simulink library "Battery_Unipi"  (R2015a)
settings: Solver=ode45  StartTime=0.0  StopTime=10.0  RelTol=1e-3
values from neighbouring files (symbols this model uses):
  Bp2 = [-1.5 1.5 7.5 15 30]    [cell_model_params.mat]
  Bp3 = [10 25 35]    [cell_model_params.mat]
  Cl = [29641.7999226 11503.9720666 12184.9115516 18949.1321111 29359.7546177 54435.9445363 17320.6503567 21800.5296599 11503.1153162 8402.73024324 12724.7029394 29641.7999226 ... (165 elements, 11x3x5)]    [cell_model_params.mat]
  Cs = [1794.38328245 1972.14957342 1304.6988008 2287.34411958 1394.94057765 2574.67200441 2711.54611884 2014.87350742 1837.29877376 1461.62116074 1549.27064076 1794.38328245 ... (165 elements, 11x3x5)]    [cell_model_params.mat]
  ENTROPY = [-0.0706337258527 -0.0545791979561 -0.0419765837168 -0.0287620517654 -0.0164740504248 -0.00302559167104 0.0100496853907 0.0236819820108 0.0382890628579 0.050946575251 0.063604087644 0.0768186195953 ... (50 elements, 50x1)]    [entropy.mat]
  N = 12    [cell_model_params.mat]
  ocv = [3.27067654763 3.32006132767 3.3625409396 3.37864461563 3.39474829166 3.41085196769 3.42695564372 3.44305931975 3.45916299578 3.4752666718 3.49137034783 3.50747402386 ... (101 elements, 1x101)]    [cell_model_params.mat]
  params_bp = [0 10 20 30 40 50 60 70 80 90 100]    [cell_model_params.mat]
  Rl = [0.00306579121698 0.00985095179058 0.015159872699 0.00697344374496 0.00685050473095 0.0168286148563 0.028842238204 0.00933556048236 0.00984564396619 0.0207825421227 0.0597713059702 0.00306579121698 ... (165 elements, 11x3x5)]    [cell_model_params.mat]
  Rs = [0.00681237649308 0.0137907776578 0.0142248736573 0.00670636858043 0.0102913336279 0.0171112771524 0.00861470287808 0.00777637938451 0.0115325080228 0.0160739212772 0.0270265485557 0.00681237649308 ... (165 elements, 11x3x5)]    [cell_model_params.mat]
  soc_bp = [0 1 2 3 4 5 6 7 8 9 10 11 ... (101 elements, 1x101)]    [cell_model_params.mat]
  SOC_EN = [0.199345854552 0.208169800236 0.215033250515 0.222873277857 0.22973569152 0.236601928766 0.244441497278 0.252282901109 0.26012751675 0.267965708772 0.275803900794 0.283643928136 ... (50 elements, 50x1)]    [entropy.mat]
undefined symbols (not defined in the file or in its folder): Cth, Ro, Rthca, Rthcc, SoC0, Ta
undefined symbols (not defined in the file): Qbattery, R0, SoCinitlut
libraries: simulink x18, Battery_Unipi x7, simulink_extras x2
settings Model: Creator=Rocco  LastModifiedBy=pc2

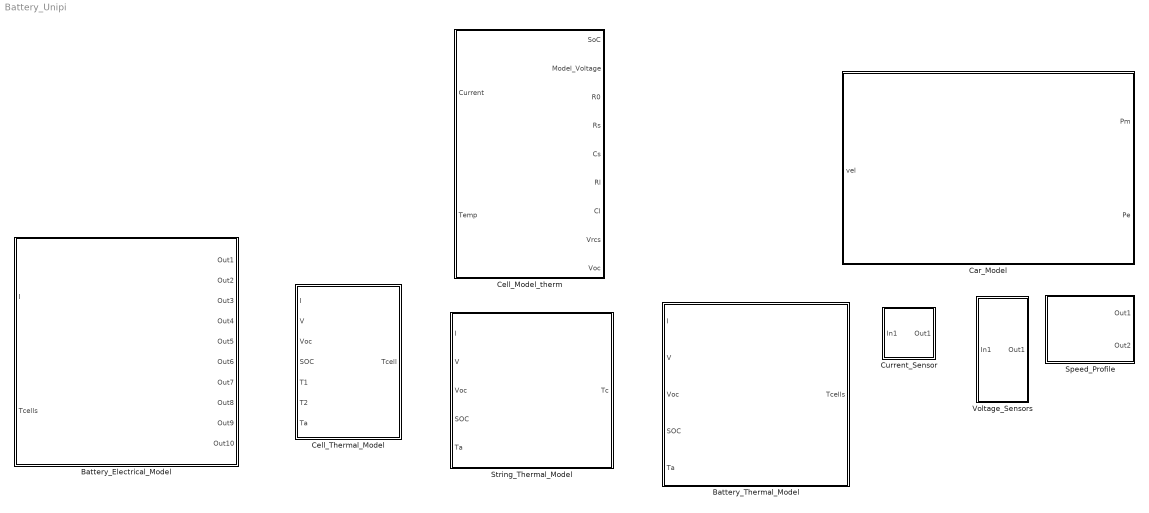
== system Battery_Unipi ==
  Battery_Electrical_Model : Subsystem  AncestorBlock=Battery_Unipi/Battery_Model_2  TreatAsAtomicUnit=on  mask{N=N, sampletime=sampletime, Qbattery=Qbattery, ocv=ocv, soc_bp=soc_bp, params_bp=params_bp, Ro=[repmat(R0,1,N)], Rs=[repmat(Rs,1,N)], Cs=[repmat(Cs,1,N)], Rl=[repmat(Rl,1,N)], Cl=[repmat(Cl,1,N)], SoC0=SoCinitlut, Bp2=Bp2, Bp3=Bp3}
      mask prompts: N "Number of cells"; sampletime "Sample time"; Qbattery "Battery Capacity (Coulomb)"; ocv "OCV-SOC LUT (101 points)"; soc_bp "OCV-SOC brakpoint (101points)"; params_bp "Parameter breackpoint (11 points)"; Ro "R0 (11 points)"; Rs "Rs (11 points)"; Cs "Cs (11 points)"; Rl "Rl (11 points)"; Cl "Cl (11 points)"; SoC0 "Initial SoC (%)"; Bp2 "Current breakpoint"; Bp3 "Temperature breakpoint"
      mask DialogControl DescTextVar Prompt: Battery composed of N series-connected cells. Each cell is modelled with an electric equivalent circuit with two RC groups. See Cell_Model block for more informations.
      mask DialogControl Control2 Prompt: Note: The OCV-SOC curve is the same for each cell.
      mask Display:
      | image('2013-9-3-5-7-21.jpg')
      | port_label('output', 1, 'SoCs')
      | port_label('output', 2, 'V_cells')
      | port_label('output', 3, 'R0')
      | port_label('output', 4, 'Rs')
      | port_label('output', 5, 'Cs')
      | port_label('output', 6, 'Rl')
      | port_label('output', 7, 'Cl')
      | port_label('output', 8, 'Vrcs')
      | port_label('output', 9, 'Voc')
      | port_label('output', 10, 'Vmcont')
      | port_label('input', 1, 'Current')
      | port_label('input', 2, 'Tcells')
  Battery_Thermal_Model : Subsystem  AncestorBlock=Battery_Unipi/Battery_Thermal_Model_obsolete  TreatAsAtomicUnit=on  mask{M=12, Rthca=Rthca, Rthcc=Rthcc, Cth=Cth, Ta=Ta, sampletime=sampletime}
      mask prompts: M "Number of cells into the string"; Rthca "Thermal resistance cell-to-ambient [K/W]"; Rthcc "Thermal resistance cell-to-cell [K/W]"; Cth "Thermal capacitance [J/W]"; Ta "Initial temperature [°C]"; sampletime "Sampletime [s]"
      mask DialogControl DescTextVar Prompt: Thermal model of a battery composed by a given number of series-connected cells, folded every M position
      mask Display:
      | image('therm.jpg')
      | port_label('output', 1, 'Tc')
      | port_label('input', 1, 'I')
      | port_label('input', 2, 'V')
      | port_label('input', 3, 'Voc')
      | port_label('input', 4, 'SOC')
      | port_label('input', 5, 'Ta')
  Car_Model : Subsystem  mask{M=1525, S=2.27, Cx=0.29, alphaR=0.01, roair=1.2, n_wheel=0.7, n_reg=0.5}
      mask prompts: M "Kerb weight (kg)"; S "Frontal area (m^2)"; Cx "Drag coefficient"; alphaR "Rolling resistance"; roair "Air density (kg m^-3)"; n_wheel "Efficiency battery->wheel"; n_reg "Efficiency wheel->battery"
      mask Display:
      | image('leaf.jpg')
      | port_label('output', 1, 'Pm')
      | port_label('output', 2, 'Pe')
      | port_label('input', 1, 'vel')
  Cell_Model_therm : Subsystem  AncestorBlock=Battery_Unipi/Cell_Model_therm  mask{Qn=Qbattery, ocv=ocv, soc_bp=soc_bp, params_bp=params_bp, R0=R0, Rs=Rs, Cs=Cs, Rl=Rl, Cl=Cl, Bp2=Bp2, Bp3=Bp3, SoC0=SoC0}
      mask prompts: Qn "Qn (Coulomb)"; ocv "OCV-SOC LUT (101 points)"; soc_bp "OCV-SOC breakpoint (101 points)"; params_bp "Parameter breakpoint (11 points)"; R0 "R0 (11 points)"; Rs "Rs (11 points)"; Cs "Cs (11 points)"; Rl "Rl (11 points)"; Cl "Cl (11 points)"; Bp2 "Current breakpoint"; Bp3 "Temperature breakpoint"; SoC0 "Initial SOC"
      mask DialogControl DescTextVar Prompt: Cell model with two RC groups
      mask Display:
      | image('unnamed.png')
      | port_label('output', 1, 'SoC')
      | port_label('output', 2, 'Vm')
      | port_label('output', 3, 'R0')
      | port_label('output', 4, 'Rs')
      | port_label('output', 5, 'Cs')
      | port_label('output', 6, 'Rl')
      | port_label('output', 7, 'Cl')
      | port_label('output', 8, 'Vrcs')
      | port_label('output', 9, 'Voc')
      | port_label('input', 1, 'Current')
      | port_label('input', 2, 'Temp')
  Cell_Thermal_Model : Subsystem  AncestorBlock=Battery_Unipi/cell_thermal_model  mask{Rthca=Rthca, Rthcc=Rthcc, Cth=Cth, Ta=24.833}
      mask prompts: Rthca "Thermal resistance cell-to-ambient [K/W]"; Rthcc "Thermal resistance cell-to-cell [K/W]"; Cth "Thermal capacitance [J/W]"; Ta "Initial temperature [°C]"
      mask Display:
      | image('big.png')
      | port_label('input', 1, 'I')
      | port_label('input', 2, 'V')
      | port_label('input', 3, 'Voc')
      | port_label('input', 4, 'SOC')
      | port_label('input', 5, 'T1')
      | port_label('input', 6, 'T2')
      | port_label('input', 7, 'Ta')
      | port_label('output', 1, 'Tc')
  Current_Sensor : Subsystem  mask{sampletime=sampletime, noisevariance=1, Offset=0, Nbits=16, FS=100}
      mask prompts: sampletime "Sample Time"; noisevariance "Variance"; Nbits "Number of bits"; FS "Full scale"
      mask DialogControl DescTextVar Prompt: This block is used to model the noise introduced by the current sensor and the ADC conversion
      mask Display: image('current_sensor.jpg')
  Speed_Profile : Subsystem  mask{selector=1}
      mask prompts: selector "Speed Profile"
      mask DialogControl DescTextVar Prompt: Select the speed test profile (1 for UDDS, 2 for HWFET, 3 for FTP, 4 for ECE_R15, 5 for EUDC, 6 for NEDC, 7 for WLTP_class_3, 8 for ArtUrban, 9 for ArtRoad, 10 for ArtMw130, 11 for ArtMw150, 12 for IM240, 13 for LA92, 14 for LA92short, 15 for NYCC, 16 for SFTP_SC03, 17 for SFTP_US06 and 18 for J1015).
      mask Display:
      | port_label('output', 1, 'Speed (km/h)')
      | port_label('output', 2, 'Speed (m/s)')
  String_Thermal_Model : Subsystem  AncestorBlock=Battery_Unipi/String_Thermal_Model_obsolete  mask{N=N, Rthca=Rthca, Rthcc=Rthcc, Cth=Cth, Ta=Ta, sampletime=sampletime}
      mask prompts: N "Number of cells"; Rthca "Thermal resistance cell-to-ambient [K/W]"; Rthcc "Thermal resistance cell-to-cell [K/W]"; Cth "Thermal capacitance [J/W]"; Ta "Initial temperature [°C]"; sampletime "Sampletime [s]"
      mask Display:
      | image('big_str.png')
      | port_label('output', 1, 'Tcell')
      | port_label('input', 1, 'I')
      | port_label('input', 2, 'V')
      | port_label('input', 3, 'Voc')
      | port_label('input', 4, 'SOC')
      | port_label('input', 5, 'Ta')
  Voltage_Sensors : Subsystem  mask{sampletime=0.1, noisevariance=1, Offset=0, Nbits=16, FS=5}
      mask prompts: sampletime "Sample Time"; noisevariance "Variance"; Nbits "Number of bits"; FS "Full scale"
      mask DialogControl DescTextVar Prompt: This block is used to model the noise introduced by the voltage sensor and the ADC conversion
      mask Display: image('ltc6804.jpg')

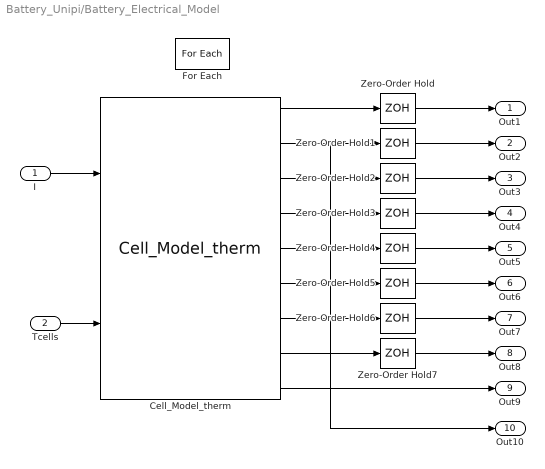
== system Battery_Unipi/Battery_Electrical_Model ==
  I : Inport  Partition=off
  Tcells : Inport  Port=2  Partition=on  PartitionDimension=1  PartitionWidth=1
  Cell_Model_therm : Battery_Unipi/Cell_Model_therm  Qn=Qbattery  ocv=ocv  soc_bp=soc_bp  params_bp=params_bp  R0=R0  Rs=Rs  Cs=Cs  Rl=Rl  Cl=Cl  Bp2=Bp2  Bp3=Bp3  SoC0=SoC0
  For Each : ForEach  DisableCoverage=on  IterateSubsysMaskParameter=off,off,on,off,off,off,on,on,on,on,on,on,off,off  SubsysMaskParameterIterationDimension=1,1,2,1,1,1,2,2,2,2,2,2,1,1  SubsysMaskParameterIterationStepSize=1,1,1,1,1,1,3,3,3,3,3,1,1,1  IndexMode=One-based
  Zero-Order Hold{,1..7} (8 alike) : ZeroOrderHold  SampleTime=sampletime
  Out1 : Outport  ConcatenationDimension=1
  Out2 : Outport  Port=2  ConcatenationDimension=1
  Out3 : Outport  Port=3  ConcatenationDimension=1
  Out4 : Outport  Port=4  ConcatenationDimension=1
  Out5 : Outport  Port=5  ConcatenationDimension=1
  Out6 : Outport  Port=6  ConcatenationDimension=1
  Out7 : Outport  Port=7  ConcatenationDimension=1
  Out8 : Outport  Port=8  ConcatenationDimension=1
  Out9 : Outport  Port=9  ConcatenationDimension=1
  Out10 : Outport  Port=10  ConcatenationDimension=1
  wires:
  Cell_Model_therm/9 -> Out9/1
  Tcells/1 -> Cell_Model_therm/2
  I/1 -> Cell_Model_therm/1
  Zero-Order Hold/1 -> Out1/1
  Cell_Model_therm/1 -> Zero-Order Hold/1
  Zero-Order Hold2/1 -> Out3/1
  Cell_Model_therm/3 -> Zero-Order Hold2/1
  Cell_Model_therm/2 -> Zero-Order Hold1/1, Out10/1
  Zero-Order Hold1/1 -> Out2/1
  Cell_Model_therm/7 -> Zero-Order Hold6/1
  Zero-Order Hold6/1 -> Out7/1
  Zero-Order Hold5/1 -> Out6/1
  Zero-Order Hold4/1 -> Out5/1
  Zero-Order Hold3/1 -> Out4/1
  Cell_Model_therm/4 -> Zero-Order Hold3/1
  Cell_Model_therm/5 -> Zero-Order Hold4/1
  Cell_Model_therm/6 -> Zero-Order Hold5/1
  Cell_Model_therm/8 -> Zero-Order Hold7/1
  Zero-Order Hold7/1 -> Out8/1

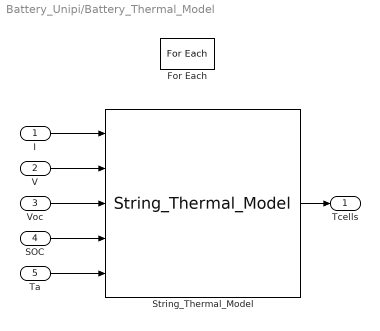
== system Battery_Unipi/Battery_Thermal_Model ==
  I : Inport  Partition=off
  V : Inport  Port=2  Partition=on  PartitionDimension=1  PartitionWidth=M
  Voc : Inport  Port=3  Partition=on  PartitionDimension=1  PartitionWidth=M
  SOC : Inport  Port=4  Partition=on  PartitionDimension=1  PartitionWidth=M
  Ta : Inport  Port=5  Partition=off
  For Each : ForEach  DisableCoverage=on  IndexMode=One-based
  String_Thermal_Model : Battery_Unipi/String_Thermal_Model  N=M  Rthca=Rthca  Rthcc=Rthcc  Cth=Cth  Ta=Ta  sampletime=sampletime
  Tcells : Outport  ConcatenationDimension=1
  wires:
  Ta/1 -> String_Thermal_Model/5
  V/1 -> String_Thermal_Model/2
  I/1 -> String_Thermal_Model/1
  String_Thermal_Model/1 -> Tcells/1
  Voc/1 -> String_Thermal_Model/3
  SOC/1 -> String_Thermal_Model/4

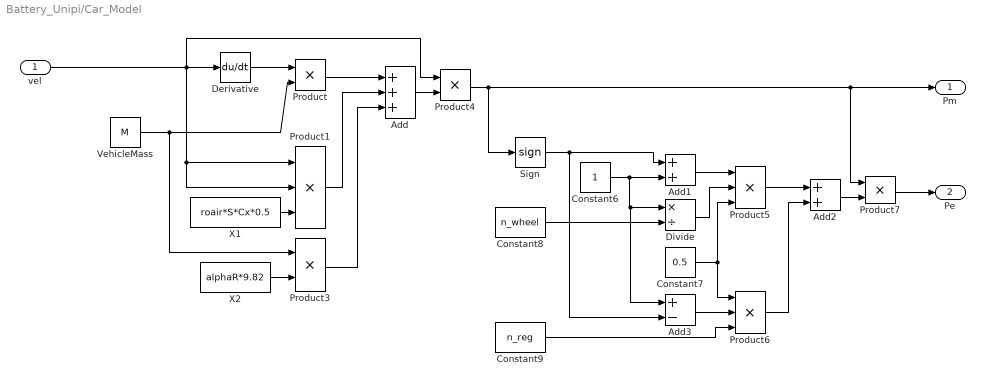
== system Battery_Unipi/Car_Model ==
  vel : Inport
  Add : Sum  Inputs=+++
  Add1 : Sum
  Add2 : Sum
  Add3 : Sum  Inputs=+-
  Constant6 : Constant
  Constant7 : Constant  Value=0.5
  Constant8 : Constant  Value=n_wheel
  Constant9 : Constant  Value=n_reg
  Derivative : Derivative
  Divide : Product  Inputs=*/
  Product{,3..4,7} (4 alike) : Product
  Product1 : Product  Inputs=3
  Product5 : Product  Inputs=3
  Product6 : Product  Inputs=3
  Sign : Signum  ZeroCross=off
  VehicleMass : Constant  Value=M
  X1 : Constant  Value=roair*S*Cx*0.5
  X2 : Constant  Value=alphaR*9.82
  Pm : Outport
  Pe : Outport  Port=2
  wires:
  Constant9/1 -> Product6/3
  Product/1 -> Add/1
  Add2/1 -> Product7/2
  Add3/1 -> Product6/2
  vel/1 -> Product4/1, Product1/2, Product1/1, Derivative/1
  VehicleMass/1 -> Product/2, Product3/1
  Product7/1 -> Pe/1
  Product3/1 -> Add/3
  Add/1 -> Product4/2
  Product5/1 -> Add2/1
  Constant7/1 -> Product6/1, Product5/3
  X2/1 -> Product3/2
  Add1/1 -> Product5/1
  Product4/1 -> Sign/1, Pm/1, Product7/1
  Sign/1 -> Add3/2, Add1/1
  Constant8/1 -> Divide/2
  Divide/1 -> Product5/2
  Product1/1 -> Add/2
  Constant6/1 -> Add3/1, Divide/1, Add1/2
  Derivative/1 -> Product/1
  Product6/1 -> Add2/2
  X1/1 -> Product1/3

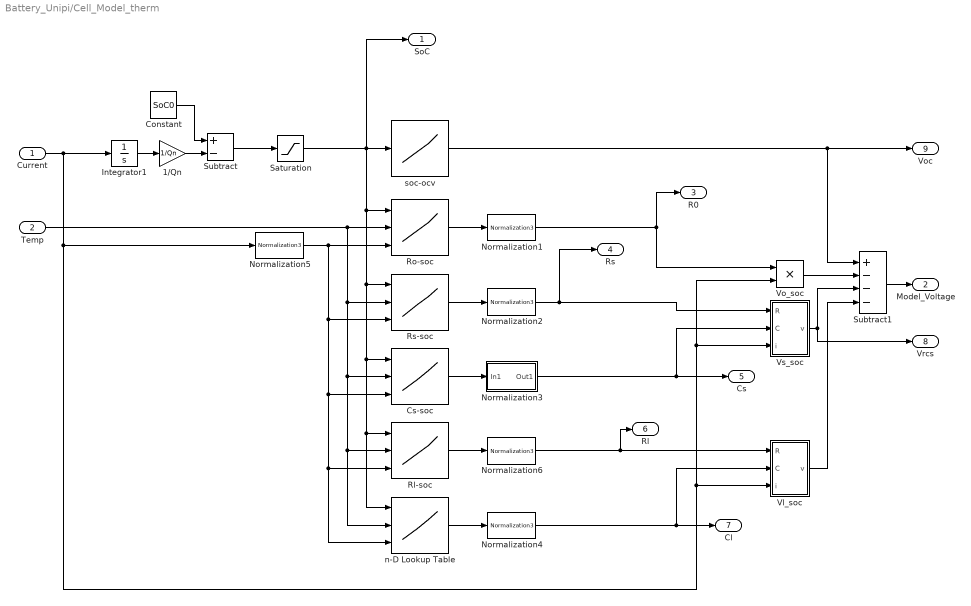
== system Battery_Unipi/Cell_Model_therm ==
  Current : Inport
  Temp : Inport  Port=2
  1/Qn : Gain  Gain=1/Qn
  Constant : Constant  Value=SoC0
  Cs-soc : Lookup_n-D  NumberOfTableDimensions=3  BreakpointsForDimension1=params_bp  BreakpointsForDimension2=Bp3  BreakpointsForDimension3=Bp2  Table=Cs  InterpMethod=Cubic spline  ExtrapMethod=Clip  UseLastTableValue=on  InternalRulePriority=Speed  RndMeth=Simplest  InputSameDT=on
  Integrator1 : Integrator
  Normalization1 : Battery_Unipi/Cell_Model_therm/Normalization3
      link override Constant3: Value=(1.5*3600)/Qn
  Normalization2 : Battery_Unipi/Cell_Model_therm/Normalization3
      link override Constant3: Value=(1.5*3600)/Qn
  Normalization3 : Subsystem  AncestorBlock=Battery_Unipi/Cell_Model/Normalization
  Normalization4 : Battery_Unipi/Cell_Model_therm/Normalization3
  Normalization5 : Battery_Unipi/Cell_Model_therm/Normalization3
      link override Constant3: Value=1.5/(Qn/3600)
  Normalization6 : Battery_Unipi/Cell_Model_therm/Normalization3
      link override Constant3: Value=(1.5*3600)/Qn
  Rl-soc : Lookup_n-D  NumberOfTableDimensions=3  BreakpointsForDimension1=params_bp  BreakpointsForDimension2=Bp3  BreakpointsForDimension3=Bp2  Table=Rl  InterpMethod=Cubic spline  ExtrapMethod=Clip  UseLastTableValue=on  InternalRulePriority=Speed  RndMeth=Simplest  InputSameDT=on
  Ro-soc : Lookup_n-D  NumberOfTableDimensions=3  BreakpointsForDimension1=params_bp  BreakpointsForDimension2=Bp3  BreakpointsForDimension3=Bp2  Table=Ro  InterpMethod=Cubic spline  ExtrapMethod=Clip  UseLastTableValue=on  InternalRulePriority=Speed  RndMeth=Simplest  InputSameDT=on
  Rs-soc : Lookup_n-D  NumberOfTableDimensions=3  BreakpointsForDimension1=params_bp  BreakpointsForDimension2=Bp3  BreakpointsForDimension3=Bp2  Table=Rs  InterpMethod=Cubic spline  ExtrapMethod=Clip  UseLastTableValue=on  InternalRulePriority=Speed  RndMeth=Simplest  InputSameDT=on
  Saturation : Saturate  UpperLimit=100  LowerLimit=0
  Subtract : Sum  Inputs=+-
  Subtract1 : Sum  Inputs=+---
  Vl_soc : Subsystem
  Vo_soc : Product
  Vs_soc : Subsystem
  n-D Lookup Table : Lookup_n-D  NumberOfTableDimensions=3  BreakpointsForDimension1=params_bp  BreakpointsForDimension2=Bp3  BreakpointsForDimension3=Bp2  Table=Cl  InterpMethod=Cubic spline  ExtrapMethod=Clip  UseLastTableValue=on  InternalRulePriority=Speed  RndMeth=Simplest  InputSameDT=on
  soc-ocv : Lookup_n-D  NumberOfTableDimensions=1  BreakpointsForDimension1=soc_bp  Table=ocv  InternalRulePriority=Speed  RndMeth=Simplest  InputSameDT=on
  SoC : Outport
  Model_Voltage : Outport  Port=2
  R0 : Outport  Port=3
  Rs : Outport  Port=4
  Cs : Outport  Port=5
  Rl : Outport  Port=6
  Cl : Outport  Port=7
  Vrcs : Outport  Port=8
  Voc : Outport  Port=9
  wires:
  Current/1 -> Integrator1/1, Normalization5/1, Vl_soc/3(i), Vs_soc/3(i), Vo_soc/2
  Normalization4/1 -> Vl_soc/2("C "), Cl/1
  Normalization3/1(Out1) -> Vs_soc/2("C "), Cs/1
  Normalization6/1 -> Vl_soc/1(R), Rl/1
  Normalization2/1 -> Vs_soc/1(R), Rs/1
  Normalization1/1 -> R0/1, Vo_soc/1
  Temp/1 -> Ro-soc/2, Rs-soc/2, n-D Lookup Table/2, Rl-soc/2, Cs-soc/2
  Subtract1/1 -> Model_Voltage/1
  Vo_soc/1 -> Subtract1/2
  Subtract/1 -> Saturation/1
  Constant/1 -> Subtract/1
  Vl_soc/1(v) -> Subtract1/4
  Vs_soc/1(v) -> Subtract1/3, Vrcs/1
  soc-ocv/1 -> Subtract1/1, Voc/1
  Rs-soc/1 -> Normalization2/1
  n-D Lookup Table/1 -> Normalization4/1
  Rl-soc/1 -> Normalization6/1
  Ro-soc/1 -> Normalization1/1
  Integrator1/1 -> 1/Qn/1
  Cs-soc/1 -> Normalization3/1(In1)
  1/Qn/1 -> Subtract/2
  Saturation/1 -> Ro-soc/1, Rs-soc/1, Cs-soc/1, Rl-soc/1, n-D Lookup Table/1, SoC/1, soc-ocv/1
  Normalization5/1 -> Ro-soc/3, n-D Lookup Table/3, Rl-soc/3, Cs-soc/3, Rs-soc/3

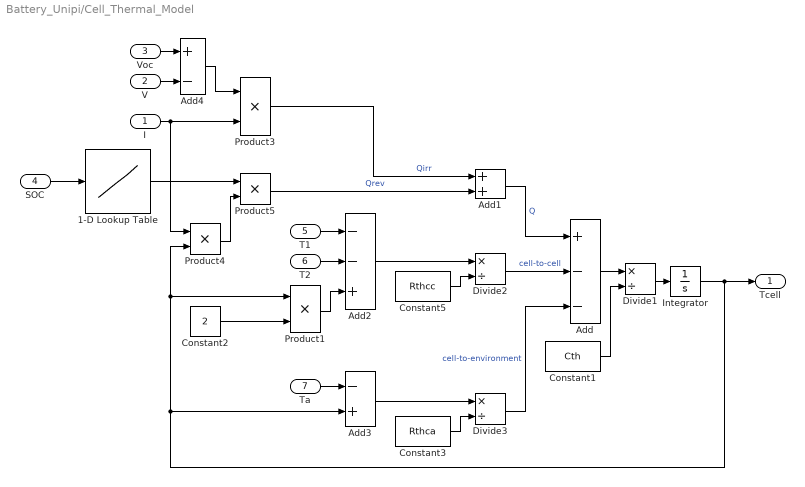
== system Battery_Unipi/Cell_Thermal_Model ==
  I : Inport
  V : Inport  Port=2
  Voc : Inport  Port=3
  SOC : Inport  Port=4
  T1 : Inport  Port=5
  T2 : Inport  Port=6
  Ta : Inport  Port=7
  1-D Lookup Table : Lookup_n-D  NumberOfTableDimensions=1  BreakpointsForDimension1=SOC_EN  BeginIndexSearchUsingPreviousIndexResult=on  Table=ENTROPY./1000  ExtrapMethod=Clip  UseLastTableValue=on  InternalRulePriority=Speed  RndMeth=Simplest  InputSameDT=on
  Add : Sum  Inputs=+--
  Add1 : Sum
  Add2 : Sum  Inputs=--+
  Add3 : Sum  Inputs=-+
  Add4 : Sum  Inputs=+-
  Constant1 : Constant  Value=Cth
  Constant2 : Constant  Value=2
  Constant3 : Constant  Value=Rthca
  Constant5 : Constant  Value=Rthcc
  Divide1 : Product  Inputs=*/
  Divide2 : Product  Inputs=*/
  Divide3 : Product  Inputs=*/
  Integrator : Integrator  InitialCondition=Ta
  Product{1,3..5} (4 alike) : Product
  Tcell : Outport
  wires:
  Integrator/1 -> Tcell/1, Product4/2, Product1/1, Add3/2
  I/1 -> Product3/2, Product4/1
  Add/1 -> Divide1/1
  Constant1/1 -> Divide1/2
  Divide1/1 -> Integrator/1
  Product4/1 -> Product5/2
  1-D Lookup Table/1 -> Product5/1
  SOC/1 -> 1-D Lookup Table/1
  Product3/1 -> Add1/1  "Qirr"
  Add1/1 -> Add/1  "Q"
  Constant2/1 -> Product1/2
  Product1/1 -> Add2/3
  T2/1 -> Add2/2
  T1/1 -> Add2/1
  Add2/1 -> Divide2/1
  Constant5/1 -> Divide2/2
  Divide2/1 -> Add/2  "cell-to-cell"
  Ta/1 -> Add3/1
  Constant3/1 -> Divide3/2
  Add3/1 -> Divide3/1
  Divide3/1 -> Add/3  "cell-to-environment"
  Product5/1 -> Add1/2  "Qrev"
  Add4/1 -> Product3/1
  Voc/1 -> Add4/1
  V/1 -> Add4/2

== system Battery_Unipi/Current_Sensor ==
  In1 : Inport
  Add : Sum
  Constant2 : Constant  Value=FS*2/(2^Nbits)
  Divide : Product  Inputs=**
  Idealized ADC quantizer : simulink_extras/Additional Discrete/Idealized ADC quantizer  NumberOfConverterBits=Nbits  Vmin=-FS  Vmax=FS  OutputDataType=single  OutputNegativeValues=on
  Noise : RandomNumber  Mean=Offset  Variance=noisevariance  SampleTime=sampletime
  Out1 : Outport
  wires:
  In1/1 -> Add/1
  Noise/1 -> Add/2
  Add/1 -> Idealized ADC quantizer/1
  Divide/1 -> Out1/1
  Idealized ADC quantizer/1 -> Divide/1
  Constant2/1 -> Divide/2

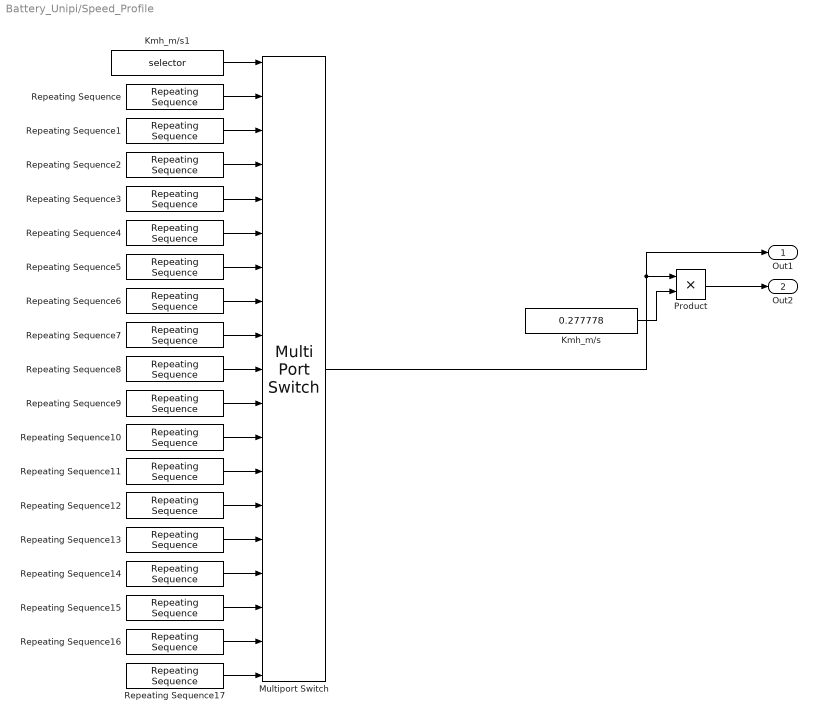
== system Battery_Unipi/Speed_Profile ==
  Kmh_m/s : Constant  Value=0.277778
  Kmh_m/s1 : Constant  Value=selector
  Multiport Switch : MultiPortSwitch  Inputs=18
  Product : Product
  Repeating Sequence : simulink/Sources/Repeating Sequence  rep_seq_t=UDDS.Time  rep_seq_y=UDDS.Data
  Repeating Sequence1 : simulink/Sources/Repeating Sequence  rep_seq_t=HWFET.Time  rep_seq_y=HWFET.Data
  Repeating Sequence10 : simulink/Sources/Repeating Sequence  rep_seq_t=ArtMw150.Time  rep_seq_y=ArtMw150.Data
  Repeating Sequence11 : simulink/Sources/Repeating Sequence  rep_seq_t=IM240.Time  rep_seq_y=IM240.Data
  Repeating Sequence12 : simulink/Sources/Repeating Sequence  rep_seq_t=LA92.Time  rep_seq_y=LA92.Data
  Repeating Sequence13 : simulink/Sources/Repeating Sequence  rep_seq_t=LA92short.Time  rep_seq_y=LA92short.Data
  Repeating Sequence14 : simulink/Sources/Repeating Sequence  rep_seq_t=NYCC.Time  rep_seq_y=NYCC.Data
  Repeating Sequence15 : simulink/Sources/Repeating Sequence  rep_seq_t=SFTP_SC03.Time  rep_seq_y=SFTP_SC03.Data
  Repeating Sequence16 : simulink/Sources/Repeating Sequence  rep_seq_t=SFTP_US06.Time  rep_seq_y=SFTP_US06.Data
  Repeating Sequence17 : simulink/Sources/Repeating Sequence  rep_seq_t=J1015.Time  rep_seq_y=J1015.Data
  Repeating Sequence2 : simulink/Sources/Repeating Sequence  rep_seq_t=FTP.Time  rep_seq_y=FTP.Data
  Repeating Sequence3 : simulink/Sources/Repeating Sequence  rep_seq_t=ECE_R15.Time  rep_seq_y=ECE_R15.Data
  Repeating Sequence4 : simulink/Sources/Repeating Sequence  rep_seq_t=EUDC.Time  rep_seq_y=EUDC.Data
  Repeating Sequence5 : simulink/Sources/Repeating Sequence  rep_seq_t=NEDC.Time  rep_seq_y=NEDC.Data
  Repeating Sequence6 : simulink/Sources/Repeating Sequence  rep_seq_t=WLTP_class_3.Time  rep_seq_y=WLTP_class_3.Data
  Repeating Sequence7 : simulink/Sources/Repeating Sequence  rep_seq_t=ArtUrban.Time  rep_seq_y=ArtUrban.Data
  Repeating Sequence8 : simulink/Sources/Repeating Sequence  rep_seq_t=ArtRoad.Time  rep_seq_y=ArtRoad.Data
  Repeating Sequence9 : simulink/Sources/Repeating Sequence  rep_seq_t=ArtMw130.Time  rep_seq_y=ArtMw130.Data
  Out1 : Outport
  Out2 : Outport  Port=2
  wires:
  Kmh_m/s1/1 -> Multiport Switch/1
  Repeating Sequence/1 -> Multiport Switch/2
  Repeating Sequence1/1 -> Multiport Switch/3
  Repeating Sequence2/1 -> Multiport Switch/4
  Repeating Sequence3/1 -> Multiport Switch/5
  Repeating Sequence4/1 -> Multiport Switch/6
  Repeating Sequence5/1 -> Multiport Switch/7
  Repeating Sequence6/1 -> Multiport Switch/8
  Repeating Sequence7/1 -> Multiport Switch/9
  Repeating Sequence8/1 -> Multiport Switch/10
  Repeating Sequence9/1 -> Multiport Switch/11
  Repeating Sequence10/1 -> Multiport Switch/12
  Kmh_m/s/1 -> Product/2
  Product/1 -> Out2/1
  Multiport Switch/1 -> Product/1, Out1/1
  Repeating Sequence11/1 -> Multiport Switch/13
  Repeating Sequence12/1 -> Multiport Switch/14
  Repeating Sequence13/1 -> Multiport Switch/15
  Repeating Sequence14/1 -> Multiport Switch/16
  Repeating Sequence15/1 -> Multiport Switch/17
  Repeating Sequence16/1 -> Multiport Switch/18
  Repeating Sequence17/1 -> Multiport Switch/19

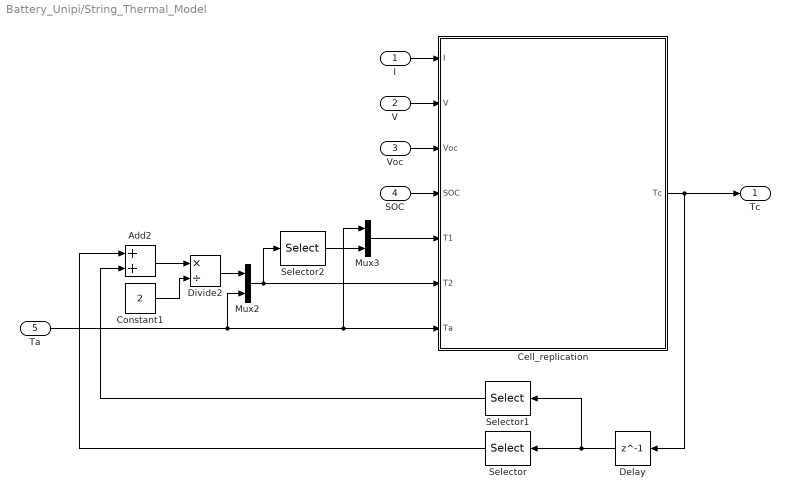
== system Battery_Unipi/String_Thermal_Model ==
  I : Inport
  V : Inport  Port=2
  Voc : Inport  Port=3
  SOC : Inport  Port=4
  Ta : Inport  Port=5
  Add2 : Sum
  Cell_replication : Subsystem  TreatAsAtomicUnit=on
  Constant1 : Constant  Value=2
  Delay : Delay  DelayLength=1  InitialCondition=0  SampleTime=sampletime
  Divide2 : Product  Inputs=*/
  Mux2 : Mux  Inputs=2
  Mux3 : Mux  Inputs=2
  Selector : Selector  NumberOfDimensions=2  InputPortWidth=N  IndexOptions=Index vector (dialog),Index vector (dialog)  Indices=[1:(N-1)],1  OutputSizes=1,1
  Selector1 : Selector  NumberOfDimensions=2  InputPortWidth=N  IndexOptions=Index vector (dialog),Index vector (dialog)  Indices=[2:N],1  OutputSizes=1,1
  Selector2 : Selector  NumberOfDimensions=2  InputPortWidth=N  IndexOptions=Index vector (dialog),Index vector (dialog)  Indices=[1:(N-1)],1  OutputSizes=1,1
  Tc : Outport
  wires:
  Delay/1 -> Selector1/1, Selector/1
  Cell_replication/1(Tc) -> Delay/1, Tc/1
  Selector/1 -> Add2/1
  V/1 -> Cell_replication/2(V)
  I/1 -> Cell_replication/1(I)
  Ta/1 -> Cell_replication/7(Ta), Mux3/1, Mux2/2
  Selector1/1 -> Add2/2
  Voc/1 -> Cell_replication/3(Voc)
  SOC/1 -> Cell_replication/4(SOC)
  Add2/1 -> Divide2/1
  Constant1/1 -> Divide2/2
  Divide2/1 -> Mux2/1
  Selector2/1 -> Mux3/2
  Mux2/1 -> Cell_replication/6(T2), Selector2/1
  Mux3/1 -> Cell_replication/5(T1)

== system Battery_Unipi/Voltage_Sensors ==
  In1 : Inport
  Add : Sum
  Constant : Constant  Value=FS/(2^Nbits)
  Divide : Product  Inputs=**
  Idealized ADC quantizer : simulink_extras/Additional Discrete/Idealized ADC quantizer  NumberOfConverterBits=Nbits  Vmin=0  Vmax=FS  OutputDataType=single  OutputNegativeValues=off
  Noise : RandomNumber  Mean=Offset  Variance=noisevariance  SampleTime=sampletime
  Out1 : Outport
  wires:
  In1/1 -> Add/1
  Noise/1 -> Add/2
  Idealized ADC quantizer/1 -> Divide/1
  Constant/1 -> Divide/2
  Add/1 -> Idealized ADC quantizer/1
  Divide/1 -> Out1/1

== system Battery_Unipi/Cell_Model_therm/Normalization3 ==
  In1 : Inport
  Constant3 : Constant  Value=(Qn/3600)/1.5
  Vo_soc1 : Product
  Out1 : Outport
  wires:
  Constant3/1 -> Vo_soc1/2
  Vo_soc1/1 -> Out1/1
  In1/1 -> Vo_soc1/1

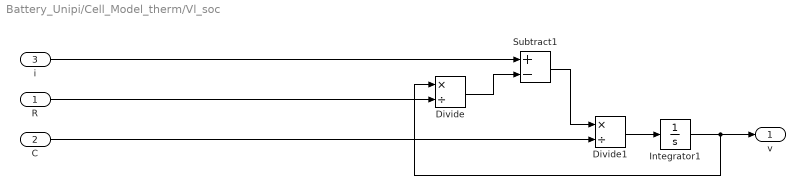
== system Battery_Unipi/Cell_Model_therm/Vl_soc ==
  R : Inport
  "C " : Inport  Port=2
  i : Inport  Port=3
  Divide : Product  Inputs=*/
  Divide1 : Product  Inputs=*/
  Integrator1 : Integrator  ContinuousStateAttributes='x1'
  Subtract1 : Sum  Inputs=+-
  v : Outport
  wires:
  "C "/1 -> Divide1/2
  R/1 -> Divide/2
  i/1 -> Subtract1/1
  Integrator1/1 -> v/1, Divide/1
  Divide1/1 -> Integrator1/1
  Subtract1/1 -> Divide1/1
  Divide/1 -> Subtract1/2

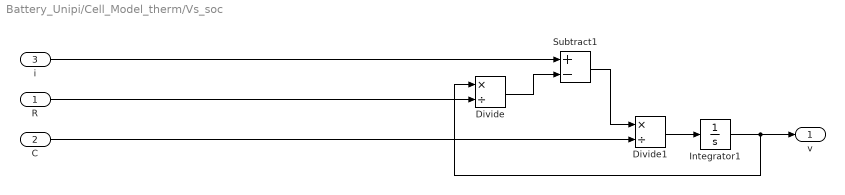
== system Battery_Unipi/Cell_Model_therm/Vs_soc ==
  R : Inport
  "C " : Inport  Port=2
  i : Inport  Port=3
  Divide : Product  Inputs=*/
  Divide1 : Product  Inputs=*/
  Integrator1 : Integrator
  Subtract1 : Sum  Inputs=+-
  v : Outport
  wires:
  R/1 -> Divide/2
  "C "/1 -> Divide1/2
  Integrator1/1 -> v/1, Divide/1
  Divide1/1 -> Integrator1/1
  Subtract1/1 -> Divide1/1
  i/1 -> Subtract1/1
  Divide/1 -> Subtract1/2

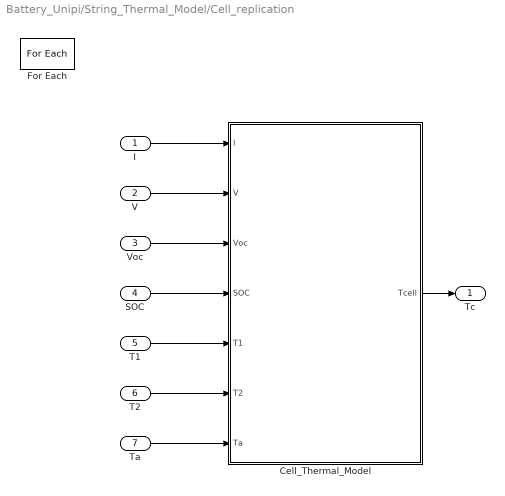
== system Battery_Unipi/String_Thermal_Model/Cell_replication ==
  I : Inport  Partition=off
  V : Inport  Port=2  Partition=on  PartitionDimension=1  PartitionWidth=1
  Voc : Inport  Port=3  Partition=on  PartitionDimension=1  PartitionWidth=1
  SOC : Inport  Port=4  Partition=on  PartitionDimension=1  PartitionWidth=1
  T1 : Inport  Port=5  Partition=on  PartitionDimension=1  PartitionWidth=1
  T2 : Inport  Port=6  Partition=on  PartitionDimension=1  PartitionWidth=1
  Ta : Inport  Port=7  Partition=off
  Cell_Thermal_Model : Subsystem  AncestorBlock=Battery_Unipi/cell_thermal_model  mask{Rthca=Rthca, Rthcc=Rthcc, Cth=Cth, Ta=Ta}
      mask prompts: Rthca "Thermal resistance cell-to-ambient [K/W]"; Rthcc "Thermal resistance cell-to-cell [K/W]"; Cth "Thermal capacitance [J/W]"; Ta "Initial temperature [°C]"
      mask Display:
      | image('big.png')
      | port_label('input', 1, 'I')
      | port_label('input', 2, 'V')
      | port_label('input', 3, 'Voc')
      | port_label('input', 4, 'SOC')
      | port_label('input', 5, 'T1')
      | port_label('input', 6, 'T2')
      | port_label('input', 7, 'Ta')
      | port_label('output', 1, 'Tc')
  For Each : ForEach  DisableCoverage=on  IndexMode=One-based
  Tc : Outport  ConcatenationDimension=1
  wires:
  T2/1 -> Cell_Thermal_Model/6(T2)
  T1/1 -> Cell_Thermal_Model/5(T1)
  Ta/1 -> Cell_Thermal_Model/7(Ta)
  V/1 -> Cell_Thermal_Model/2(V)
  I/1 -> Cell_Thermal_Model/1(I)
  Cell_Thermal_Model/1(Tcell) -> Tc/1
  Voc/1 -> Cell_Thermal_Model/3(Voc)
  SOC/1 -> Cell_Thermal_Model/4(SOC)

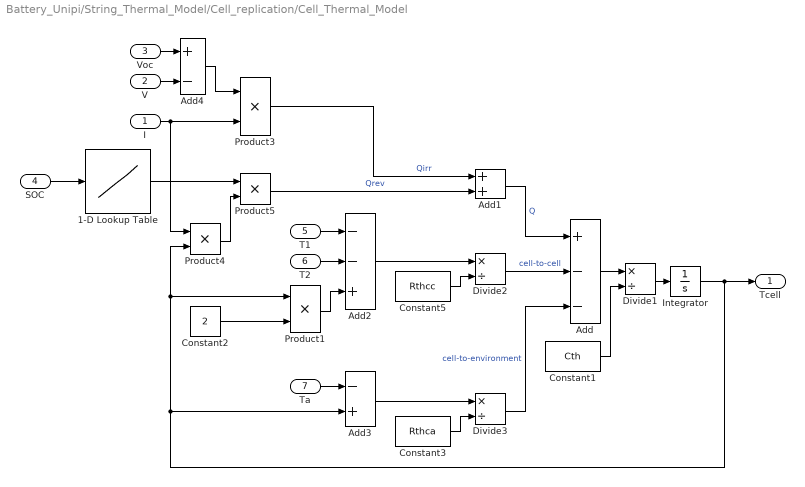
== system Battery_Unipi/String_Thermal_Model/Cell_replication/Cell_Thermal_Model ==
  I : Inport
  V : Inport  Port=2
  Voc : Inport  Port=3
  SOC : Inport  Port=4
  T1 : Inport  Port=5
  T2 : Inport  Port=6
  Ta : Inport  Port=7
  1-D Lookup Table : Lookup_n-D  NumberOfTableDimensions=1  BreakpointsForDimension1=SOC_EN.*100  Table=ENTROPY./1000  ExtrapMethod=Clip  UseLastTableValue=on  InternalRulePriority=Speed  RndMeth=Simplest  InputSameDT=on
  Add : Sum  Inputs=+--
  Add1 : Sum
  Add2 : Sum  Inputs=--+
  Add3 : Sum  Inputs=-+
  Add4 : Sum  Inputs=+-
  Constant1 : Constant  Value=Cth
  Constant2 : Constant  Value=2
  Constant3 : Constant  Value=Rthca
  Constant5 : Constant  Value=Rthcc
  Divide1 : Product  Inputs=*/
  Divide2 : Product  Inputs=*/
  Divide3 : Product  Inputs=*/
  Integrator : Integrator  InitialCondition=Ta
  Product{1,3..5} (4 alike) : Product
  Tcell : Outport
  wires:
  Integrator/1 -> Tcell/1, Product4/2, Product1/1, Add3/2
  I/1 -> Product3/2, Product4/1
  Add/1 -> Divide1/1
  Constant1/1 -> Divide1/2
  Divide1/1 -> Integrator/1
  Product4/1 -> Product5/2
  1-D Lookup Table/1 -> Product5/1
  SOC/1 -> 1-D Lookup Table/1
  Product3/1 -> Add1/1  "Qirr"
  Add1/1 -> Add/1  "Q"
  Constant2/1 -> Product1/2
  Product1/1 -> Add2/3
  T2/1 -> Add2/2
  T1/1 -> Add2/1
  Add2/1 -> Divide2/1
  Constant5/1 -> Divide2/2
  Divide2/1 -> Add/2  "cell-to-cell"
  Ta/1 -> Add3/1
  Constant3/1 -> Divide3/2
  Add3/1 -> Divide3/1
  Divide3/1 -> Add/3  "cell-to-environment"
  Product5/1 -> Add1/2  "Qrev"
  Add4/1 -> Product3/1
  V/1 -> Add4/2
  Voc/1 -> Add4/1
